simulink model "symulacja"  (R2017a)
settings: Solver=ode23  StartTime=0  StopTime=50  MaxStep=0.0001  RelTol=1e-3  EnableMultiTasking=on
undefined symbols (not defined in the file): In, J, Kp, Kt, Kw, lambda_n, m, psi_e, R, T, TR, Uz0, V, wz, Y
libraries: powerlib x1
settings Model: Creator=Admin  LastModifiedBy=Kuba
settings DataIOCC: SaveFormat=StructureWithTime  SignalLoggingSaveFormat=ModelDataLogs
settings OptimizationCC: LifeSpan=inf
settings DebuggingCC: MultiTaskDSMMsg=warning  MultiTaskCondExecSysMsg=none  SFUnexpectedBacktrackingDiag=warning  SFNoUnconditionalDefaultTransitionDiag=warning  SFExecutionAtInitializationDiag=none
settings HardwareCC: ProdBitPerSizeT=32  ProdBitPerPtrDiffT=32  ProdWordSize=32  ProdHWDeviceType=Specified
settings GRTTargetCC: TargetLangStandard=C89/C90 (ANSI)  GeneratePreprocessorConditionals=Disable all
settings ConfigComp: CovMetricSettings=dw  CovHtmlReporting=on  CovSaveCumulativeToWorkspaceVar=on  CovSaveSingleToWorkspaceVar=on  CovExternalEMLEnable=off

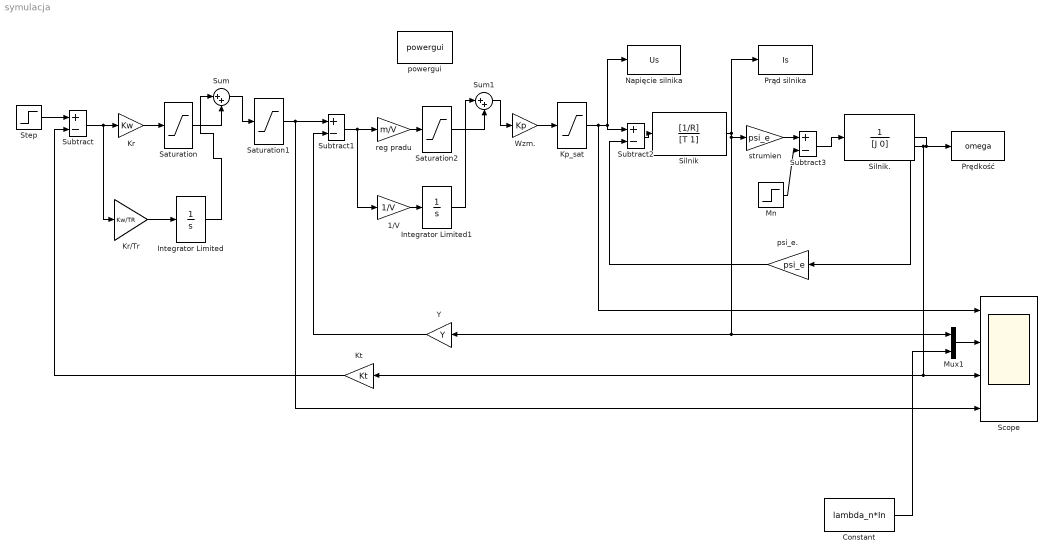
== system symulacja ==
  1/V : Gain  Gain=1/V
  Constant : Constant  Value=lambda_n*In
  Integrator Limited : Integrator  LimitOutput=on  UpperSaturationLimit=10  LowerSaturationLimit=-10
  Integrator Limited1 : Integrator  LimitOutput=on  UpperSaturationLimit=10  LowerSaturationLimit=-10
  Kp_sat : Saturate  UpperLimit=500  LowerLimit=-500
  Kr : Gain  Gain=Kw
  Kr/Tr : Gain  Gain=Kw/TR
  Kt : Gain  Gain=Kt
  Mn : Step  After=0  SampleTime=0
  Mux1 : Mux  Inputs=2
  Napięcie silnika : ToWorkspace  VariableName=Us  SaveFormat=Structure With Time  SampleTime=-1
  Prąd silnika : ToWorkspace  VariableName=Is  SaveFormat=Structure With Time  SampleTime=-1
  Prędkość : ToWorkspace  VariableName=omega  SaveFormat=Structure With Time  SampleTime=-1
  Saturation : Saturate  UpperLimit=10  LowerLimit=-10
  Saturation1 : Saturate  UpperLimit=Uz0  LowerLimit=-Uz0
  Saturation2 : Saturate  UpperLimit=10  LowerLimit=-10
  Scope : Scope  NumInputPorts=4
  Silnik : TransferFcn  Numerator=[1/R]  Denominator=[T 1]
  Silnik. : TransferFcn  Denominator=[J 0]
  Step : Step  After=wz  SampleTime=0
  Subtract{,1..3} (4 alike) : Sum  Inputs=+-
  Sum : Sum  Inputs=|++
  Sum1 : Sum  Inputs=|++
  Wzm. : Gain  Gain=Kp
  Y : Gain  Gain=Y
  powergui : powerlib/powergui  Priority=1  SimulationMode=Discrete  SampleTime=2e-04  frequency=60  Iterations=50  frequencyindice=60  Pbase=100e6  ErrMax=1e-4  UnitsV=kV  UnitsW=MW  buscounter=0  FunctionMessages=off  echomessages=off  EnableUseOfTLC=off  CurrentSourceSwitches=off  DisableSnubberDevices=off  DisableRonSwitches=off  DisableVfSwitches=off  DisplayEquations=off  SolverType=Tustin  Interpol=off  ExternalGateDelay=off  methode=off  Ts=10  x0status=blocks  SPID=off  SwTol=0  HookPort=off  RestoreLinks=warning  ResistiveCurrentMeasurement=off  Frange=[0:2:500]  Ylog=off  Xlog=on  ShowGrid=off  save=off  variable=ZData  structure=0  ZoomFFT=off  StartTime=0.0  cycles=1  DisplayStyle=1  fundamental=60  FreqAxis=off  MaxFrequency=1000  frequencyindicesteady=1  RmsSteady=1  display=off
  psi_e. : Gain  Gain=psi_e
  reg pradu : Gain  Gain=m/V
  strumien : Gain  Gain=psi_e
  wires:
  Step/1 -> Subtract/1
  Kr/1 -> Saturation/1
  Subtract/1 -> Kr/Tr/1, Kr/1
  Kr/Tr/1 -> Integrator Limited/1
  Saturation1/1 -> Scope/4, Subtract1/1
  Subtract1/1 -> 1/V/1, reg pradu/1
  reg pradu/1 -> Saturation2/1
  1/V/1 -> Integrator Limited1/1
  Sum1/1 -> Wzm./1
  Wzm./1 -> Kp_sat/1
  Kp_sat/1 -> Scope/1, Subtract2/1, Napięcie silnika/1
  Subtract2/1 -> Silnik/1
  Silnik/1 -> strumien/1, Mux1/1, Y/1, Prąd silnika/1
  strumien/1 -> Subtract3/1
  Subtract3/1 -> Silnik./1
  Mn/1 -> Subtract3/2
  psi_e./1 -> Subtract2/2
  Y/1 -> Subtract1/2
  Kt/1 -> Subtract/2
  Silnik./1 -> psi_e./1, Kt/1, Scope/3, Prędkość/1
  Constant/1 -> Mux1/2
  Saturation/1 -> Sum/2
  Integrator Limited/1 -> Sum/1
  Sum/1 -> Saturation1/1
  Integrator Limited1/1 -> Sum1/1
  Saturation2/1 -> Sum1/2
  Mux1/1 -> Scope/2
